simulink model "Aula_06_12_23"  (R2022a)
settings: Solver=VariableStepAuto  StartTime=0.0  StopTime=25  RelTol=1e-3
settings Model: Creator=Aluno  LastModifiedBy=Aluno

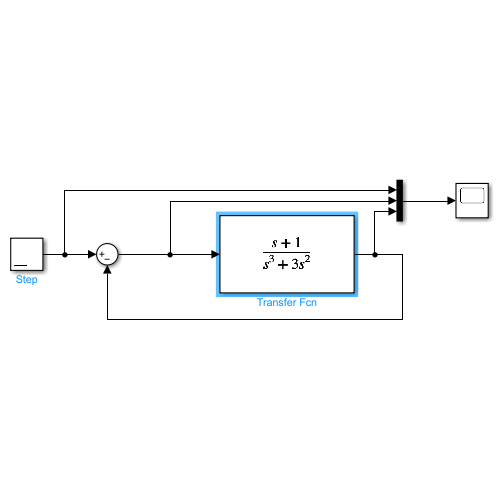
[thumbnail: Simulink's stored preview of the top-level diagram]
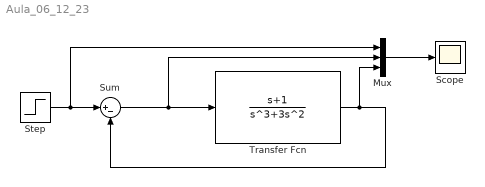
== system Aula_06_12_23 ==
  Mux : Mux  Inputs=3
  Scope : Scope
  Step : Step  SampleTime=0
  Sum : Sum  Inputs=|+-
  Transfer Fcn : TransferFcn  Numerator=[1 1]  Denominator=[1 3 0 0]
  wires:
  Transfer Fcn/1 -> Mux/3, Sum/2
  Sum/1 -> Mux/2, Transfer Fcn/1
  Step/1 -> Mux/1, Sum/1
  Mux/1 -> Scope/1
